simulink model "SDR_sample"  (Simulink 8.1)
settings: Solver=VariableStepDiscrete  StartTime=0.0  StopTime=999  RelTol=1e-3
values from neighbouring files (symbols this model uses):
  snrdB = snrdb(i)    [RunSDR.m]    (also in RunSDR_sample.m; pnorm_snrdBvsPd.m)
libraries: commchan3 x1, commdigbbndpm3 x1, commrandsrc2 x1, simulink x1
settings Model: Creator=Gaurav  LastModifiedBy=Gaurav
settings DataIOCC: SignalLoggingSaveFormat=Dataset
settings OptimizationCC: ExpressionDepthLimit=128
settings DebuggingCC: FcnCallInpInsideContextMsg=EnableAllAsError
settings GRTTargetCC: CombineOutputUpdateFcns=on  GRTInterface=off

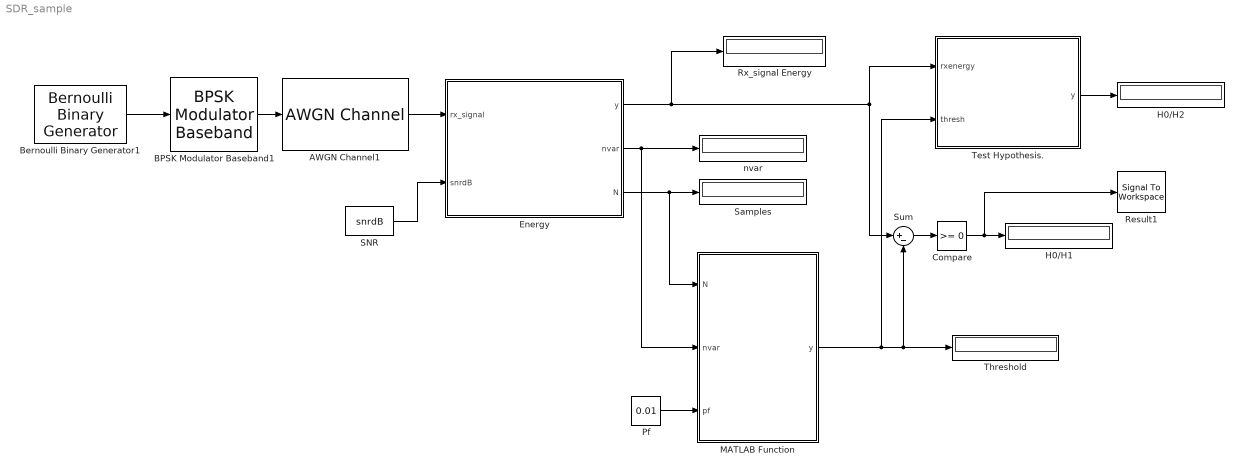
== system SDR_sample ==
  AWGN Channel1 : commchan3/AWGN Channel  InputProcessing=Columns as channels (frame based)  seed=67  noiseMode="Signal to noise ratio  (SNR)"  EbNodB=10  EsNodB=10  SNRdB=snrdB  bitsPerSym=1  Ps=1  Tsym=1  variance=1
  BPSK Modulator Baseband1 : commdigbbndpm3/BPSK Modulator Baseband  Ph=0  outDtype=double  outWordLen=16  outUDDataType=sfix(16)  outFracLenMode=Best precision  outFracLen=15
  Bernoulli Binary Generator1 : commrandsrc2/Bernoulli Binary Generator  P=0.5  seed=90  Ts=0.01  frameBased=on  sampPerFrame=100  orient=off  outDataType=double
  Compare : simulink/Logic and Bit Operations/Compare To Zero  relop=>=  OutDataTypeStr=boolean
  Energy : MATLAB Function  TreatAsAtomicUnit=on
  H0/H1 : Display
  H0/H2 : Display
  MATLAB Function : MATLAB Function  TreatAsAtomicUnit=on
  Pf : Constant  Value=0.01
  Result1 : SignalToWorkspace  VariableName=Stat
      settings: CopyFcn=dspblkcopystw(gcbh);
  Rx_signal Energy : Display
  SNR : Constant  Value=snrdB
  Samples : Display
  Sum : Sum  Inputs=|+-
  Test Hypothesis. : MATLAB Function  TreatAsAtomicUnit=on
  Threshold : Display
  nvar : Display
  wires:
  BPSK Modulator Baseband1/1 -> AWGN Channel1/1
  AWGN Channel1/1 -> Energy/1(rx_signal)
  SNR/1 -> Energy/2(snrdB)
  Energy/1(y) -> Sum/1, Test Hypothesis./1(rxenergy), Rx_signal Energy/1
  Energy/2(nvar) -> MATLAB Function/2(nvar), nvar/1
  Energy/3(N) -> MATLAB Function/1(N), Samples/1
  Pf/1 -> MATLAB Function/3(pf)
  MATLAB Function/1(y) -> Test Hypothesis./2(thresh), Threshold/1, Sum/2
  Sum/1 -> Compare/1
  Compare/1 -> Result1/1, H0/H1/1
  Test Hypothesis./1(y) -> H0/H2/1
  Bernoulli Binary Generator1/1 -> BPSK Modulator Baseband1/1

== matlab function MATLAB Function ==
  data: N input double; y output double; nvar input double; pf input double
function y = Threshold(N,nvar,pf)
    coder.extrinsic('qfuncinv');
    t=double(zeros(1,1));
    t=qfuncinv(pf);
    thresh=double(zeros(1,1));
    thresh = sqrt(2*N*nvar^4)*t+N*nvar^2;
y=thresh;

== matlab function Energy ==
  data: rx_signal input double; y output double; snrdB input double; nvar output double; N output double
function [y,nvar,N] = Energy(rx_signal,snrdB)
    [n,m]=size(rx_signal);
    %energy=double(zeros(1,1));
    energy = sum(abs(rx_signal).^2); 
    snr = 10^(snrdB/20);
    nvar = 1/snr;                               % noise variance
    y = energy;
    N=n;

== matlab function Test Hypothesis. ==
  data: rxenergy input double; y output double; thresh input double
function y = Detectionprob(rxenergy,thresh)
       t=double(zeros(1,1));
       if(rxenergy>=thresh)
           t=t+1;
       end
%     [p q]=size(R);
%     detect=double(zeros(1,1));
%     for i=1:p
%         p
%         if(R(p,1)==1)
%             detect=detect+1;
%             detect
%         end
%     end
y = t;
